simulink model "dc_motor_system"  (R2014a)
settings: Solver=ode45  StartTime=0.0  StopTime=5  RelTol=1e-3
settings Model: Creator=Divya M  LastModifiedBy=Divya M

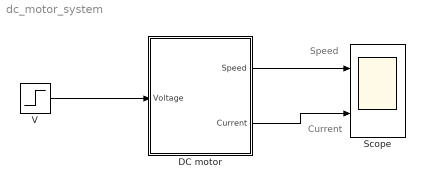
== system dc_motor_system ==
  note: Current
  note: Speed
  DC motor : Subsystem
  Scope : Scope  NumInputPorts=2
      settings: YMin=-0.01~-0.1  YMax=0.11~1.1
  V : Step  SampleTime=0
  wires:
  V/1 -> DC motor/1(Voltage)
  DC motor/1(Speed) -> Scope/1
  DC motor/2(Current) -> Scope/2

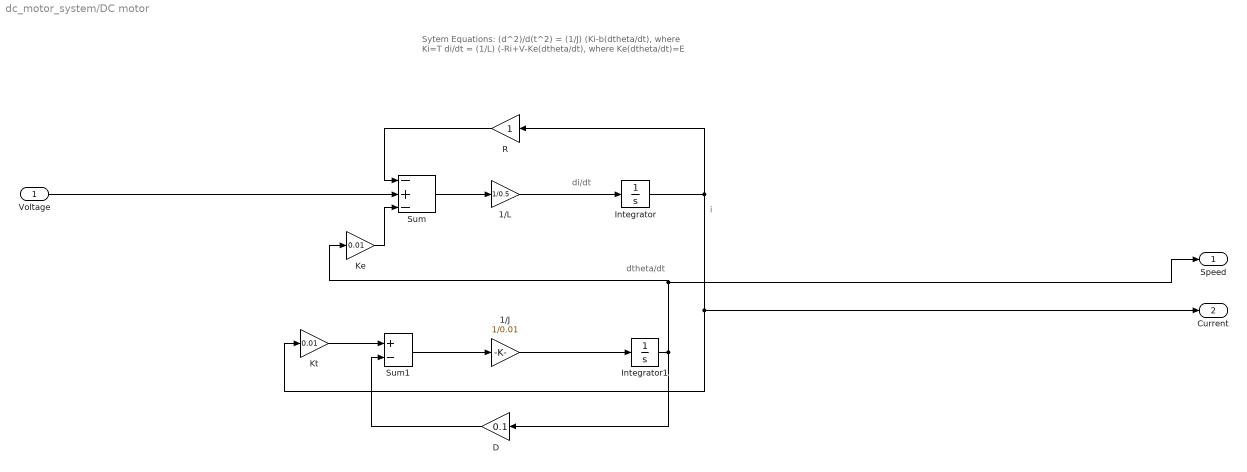
== system dc_motor_system/DC motor ==
  note: Sytem Equations:
      |
      | (d^2)/d(t^2) = (1/J) (Ki-b(dtheta/dt), where Ki=T
      | di/dt = (1/L) (-Ri+V-Ke(dtheta/dt), where Ke(dtheta/dt)=E
  note: dtheta/dt
  note: i
  note: di/dt
  Voltage : Inport
  1/J : Gain  Gain=1/0.01
  1/L : Gain  Gain=1/0.5
  D : Gain  Gain=0.1
  Integrator : Integrator
  Integrator1 : Integrator
  Ke : Gain  Gain=0.01
  Kt : Gain  Gain=0.01
  R : Gain
  Sum : Sum  Inputs=-+-
  Sum1 : Sum  Inputs=+-
  Speed : Outport
  Current : Outport  Port=2
  wires:
  Voltage/1 -> Sum/2
  1/J/1 -> Integrator1/1
  Kt/1 -> Sum1/1
  Ke/1 -> Sum/3
  Integrator1/1 -> Speed/1, Ke/1, D/1
  Integrator/1 -> R/1, Current/1, Kt/1
  Sum1/1 -> 1/J/1
  R/1 -> Sum/1
  D/1 -> Sum1/2
  Sum/1 -> 1/L/1
  1/L/1 -> Integrator/1
